simulink model "Assignment1"  (R2020a)
settings: Solver=FixedStepAuto  StartTime=0.0  StopTime=3  FixedStep=1e-3  RelTol=1e-3  EnableMultiTasking=on
undefined symbols (not defined in the file): D0, D1, D10, D11, D12, D13, D2, D3, D4, D5, D6, D7, D8, D9, PTA0, PTA1, PTA2, PTB23, PTB9, PTC16, PTC17, PTC2, PTC3, PTC4, PTD0, PTD1, PTD2, PTD3
libraries: frdmk64flib x19
settings Model: ExtModeTrigDuration=5  Creator=theodor  LastModifiedBy=theodor
settings OptimizationCC: EnhancedBackFolding=on  PassReuseOutputArgsAs=Individual arguments  ZeroExternalMemoryAtStartup=off  ZeroInternalMemoryAtStartup=off  MaxStackSize=64  OptimizeBlockOrder=speed  DifferentSizesBufferReuse=on  OptimizationCustomize=off  EfficientTunableParamExpr=on
settings DebuggingCC: ParameterTunabilityLossMsg=error
settings HardwareCC: ProdBitPerPointer=32  ProdBitPerSizeT=32  ProdBitPerPtrDiffT=32  ProdLargestAtomicInteger=Long  ProdLargestAtomicFloat=Double  ProdWordSize=32  ProdHWDeviceType=ARM Compatible->ARM Cortex
settings SFSimCC: MATLABDynamicMemAlloc=off
settings RTWCC: SystemTargetFile=ert.tlc  HardwareBoard=NXP FRDM-K64F  TemplateMakefile=ert_default_tmf  Toolchain=GNU Tools for ARM Embedded Processors
settings CodeAppCC: ForceParamTrailComments=on  IgnoreCustomStorageClasses=off  OperatorAnnotations=on  SimulinkDataObjDesc=on  SFDataObjDesc=on  InsertBlockDesc=on

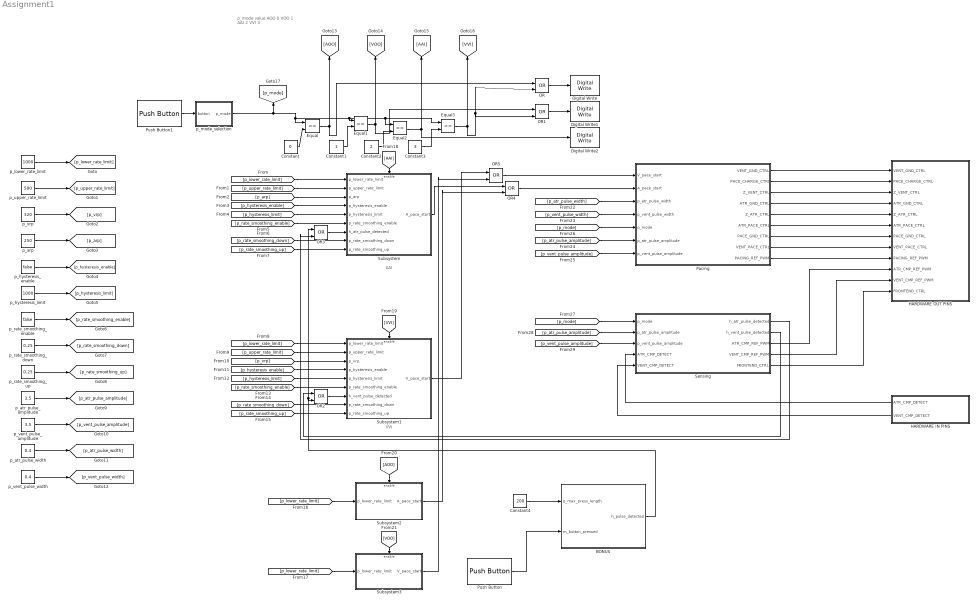
== system Assignment1 ==
  note: VVI
  note: AAI
  note: p_mode
      | value
      |
      | AOO
      | 0
      |
      | VOO
      | 1
      |
      | AAI
      | 2
      |
      | VVI
      | 3
  BONUS : Stateflow chart  TreatAsAtomicUnit=on
  Constant : Constant  Value=0
  Constant1 : Constant
  Constant2 : Constant  Value=2
  Constant3 : Constant  Value=3
  Constant4 : Constant  Value=200
  Digital Write : frdmk64flib/Digital Write  Whichpin=RED_LED
  Digital Write1 : frdmk64flib/Digital Write  Whichpin=GREEN_LED
  Digital Write2 : frdmk64flib/Digital Write  Whichpin=BLUE_LED
  Equal{,1..3} (4 alike) : RelationalOperator  Operator===  OutDataTypeStr=boolean  RndMeth=Simplest
  HARDWARE IN PINS : Subsystem
  HARDWARE OUT PINS : Subsystem
  OR{,1..5} (6 alike) : Logic  Operator=OR  IconShape=distinctive  AllPortsSameDT=off  OutDataTypeStr=boolean
  Pacing : Subsystem
  Push Button : frdmk64flib/Push Button  Whichswitch=SW3  SampleTime1=-1
  Push Button1 : frdmk64flib/Push Button  Whichswitch=SW2  SampleTime1=-1
  Sensing : Subsystem
  Subsystem : Subsystem
  Subsystem1 : Subsystem
  Subsystem2 : Subsystem
  Subsystem3 : Subsystem
  p_arp : Constant  Value=250
  p_atr_pulse_amplitude : Constant  Value=3.5
  p_atr_pulse_width : Constant  Value=0.4
  p_hysteresis_enable : Constant  Value=false
  p_hysteresis_limit : Constant  Value=1000
  p_lower_rate_limit : Constant  Value=1000
  p_mode_selection : Stateflow chart  TreatAsAtomicUnit=on
  p_rate_smoothing_down : Constant  Value=0.25
  p_rate_smoothing_enable : Constant  Value=false
  p_rate_smoothing_up : Constant  Value=0.25
  p_upper_rate_limit : Constant  Value=500
  p_vent_pulse_amplitude : Constant  Value=3.5
  p_vent_pulse_width : Constant  Value=0.4
  p_vrp : Constant  Value=320
  wires:
  Pacing/1(VENT_GND_CTRL) -> HARDWARE OUT PINS/1(VENT_GND_CTRL)
  Pacing/2(PACE_CHARGE_CTRL) -> HARDWARE OUT PINS/2(PACE_CHARGE_CTRL)
  Pacing/3(Z_VENT_CTRL) -> HARDWARE OUT PINS/3(Z_VENT_CTRL)
  Pacing/4(ATR_GND_CTRL) -> HARDWARE OUT PINS/4(ATR_GND_CTRL)
  Pacing/5(Z_ATR_CTRL) -> HARDWARE OUT PINS/5(Z_ATR_CTRL)
  Pacing/6(ATR_PACE_CTRL) -> HARDWARE OUT PINS/6(ATR_PACE_CTRL)
  Pacing/7(PACE_GND_CTRL) -> HARDWARE OUT PINS/7(PACE_GND_CTRL)
  Pacing/8(VENT_PACE_CTRL) -> HARDWARE OUT PINS/8(VENT_PACE_CTRL)
  Pacing/9(PACING_REF_PWM) -> HARDWARE OUT PINS/9(PACING_REF_PWM)
  Sensing/5(FRONTEND_CTRL) -> HARDWARE OUT PINS/12(FRONTEND_CTRL)
  Sensing/4(VENT_CMP_REF_PWM) -> HARDWARE OUT PINS/11(VENT_CMP_REF_PWM)
  Sensing/3(ATR_CMP_REF_PWM) -> HARDWARE OUT PINS/10(ATR_CMP_REF_PWM)
  HARDWARE IN PINS/1(ATR_CMP_DETECT) -> Sensing/4(ATR_CMP_DETECT)
  HARDWARE IN PINS/2(VENT_CMP_DETECT) -> Sensing/5(VENT_CMP_DETECT)
  p_mode_selection/1(p_mode) -> [p_mode], Equal3/1, Equal2/1, Equal1/1, Equal/1
  Sensing/1(h_atr_pulse_detected) -> OR3/2
  Subsystem/1(A_pace_start) -> OR4/1
  Constant/1 -> Equal/2
  Constant1/1 -> Equal1/2
  Constant2/1 -> Equal2/2
  Constant3/1 -> Equal3/2
  Equal2/1 -> Digital Write2/1, [AAI]
  Sensing/2(h_vent_pulse_detected) -> OR2/1
  Equal3/1 -> OR1/2, OR/2, [VVI]
  Equal/1 -> OR/1, [AOO]
  Equal1/1 -> OR1/1, [VOO]
  OR1/1 -> Digital Write1/1
  OR/1 -> Digital Write/1
  Push Button/1 -> BONUS/2(m_button_pressed)
  OR2/1 -> Subsystem1/7(h_vent_pulse_detected)
  BONUS/1(h_pulse_detected) -> OR3/1, OR2/2
  OR3/1 -> Subsystem/7(h_atr_pulse_detected)
  Constant4/1 -> BONUS/1(p_max_press_length)
  Push Button1/1 -> p_mode_selection/1(button)
  Subsystem2/1(A_pace_start) -> OR4/2
  OR4/1 -> Pacing/2(A_pace_start)
  Subsystem1/1(V_pace_start) -> OR5/1
  Subsystem3/1(V_pace_start) -> OR5/2
  OR5/1 -> Pacing/1(V_pace_start)
  p_lower_rate_limit/1 -> [p_lower_rate_limit]
  p_vent_pulse_width/1 -> [p_vent_pulse_width]
  p_atr_pulse_width/1 -> [p_atr_pulse_width]
  p_vent_pulse_amplitude/1 -> [p_vent_pulse_amplitude]
  p_atr_pulse_amplitude/1 -> [p_atr_pulse_amplitude]
  p_rate_smoothing_up/1 -> [p_rate_smoothing_up]
  p_rate_smoothing_down/1 -> [p_rate_smoothing_down]
  p_rate_smoothing_enable/1 -> [p_rate_smoothing_enable]
  p_hysteresis_limit/1 -> [p_hysteresis_limit]
  p_hysteresis_enable/1 -> [p_hysteresis_enable]
  p_arp/1 -> [p_arp]
  p_vrp/1 -> [p_vrp]
  p_upper_rate_limit/1 -> [p_upper_rate_limit]
  [p_lower_rate_limit] -> Subsystem/1(p_lower_rate_limit)
  [p_upper_rate_limit] -> Subsystem/2(p_upper_rate_limit)
  [p_arp] -> Subsystem/3(p_arp)
  [p_hysteresis_enable] -> Subsystem/4(p_hysteresis_enable)
  [p_hysteresis_limit] -> Subsystem/5(p_hysteresis_limit)
  [p_rate_smoothing_enable] -> Subsystem/6(p_rate_smoothing_enable)
  [p_rate_smoothing_down] -> Subsystem/8(p_rate_smoothing_down)
  [p_rate_smoothing_up] -> Subsystem/9(p_rate_smoothing_up)
  [p_lower_rate_limit] -> Subsystem1/1(p_lower_rate_limit)
  [p_upper_rate_limit] -> Subsystem1/2(p_upper_rate_limit)
  [p_vrp] -> Subsystem1/3(p_vrp)
  [p_hysteresis_enable] -> Subsystem1/4(p_hysteresis_enable)
  [p_hysteresis_limit] -> Subsystem1/5(p_hysteresis_limit)
  [p_rate_smoothing_enable] -> Subsystem1/6(p_rate_smoothing_enable)
  [p_rate_smoothing_down] -> Subsystem1/8(p_rate_smoothing_down)
  [p_rate_smoothing_up] -> Subsystem1/9(p_rate_smoothing_up)
  [p_lower_rate_limit] -> Subsystem2/1(p_lower_rate_limit)
  [p_lower_rate_limit] -> Subsystem3/1(p_lower_rate_limit)
  [AAI] -> Subsystem/Enable
  [VVI] -> Subsystem1/Enable
  [AOO] -> Subsystem2/Enable
  [VOO] -> Subsystem3/Enable
  [p_atr_pulse_width] -> Pacing/3(p_atr_pulse_width)
  [p_atr_pulse_amplitude] -> Pacing/6(p_atr_pulse_amplitude)
  [p_vent_pulse_amplitude] -> Pacing/7(p_vent_pulse_amplitude)
  [p_vent_pulse_width] -> Pacing/4(p_vent_pulse_width)
  [p_mode] -> Sensing/1(p_mode)
  [p_mode] -> Pacing/5(p_mode)
  [p_atr_pulse_amplitude] -> Sensing/2(p_atr_pulse_amplitude)
  [p_vent_pulse_amplitude] -> Sensing/3(p_vent_pulse_amplitude)

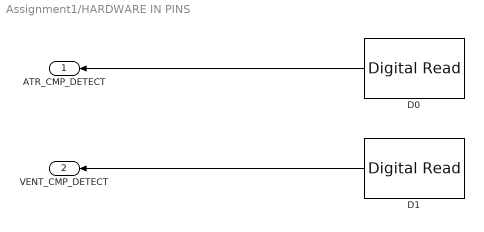
== system Assignment1/HARDWARE IN PINS ==
  D0 : frdmk64flib/Digital Read  Whichpin=PTC16 (D0)  SampleTime=-1
  D1 : frdmk64flib/Digital Read  Whichpin=PTC17 (D1)  SampleTime=-1
  ATR_CMP_DETECT : Outport
  VENT_CMP_DETECT : Outport  Port=2
  wires:
  D1/1 -> VENT_CMP_DETECT/1
  D0/1 -> ATR_CMP_DETECT/1

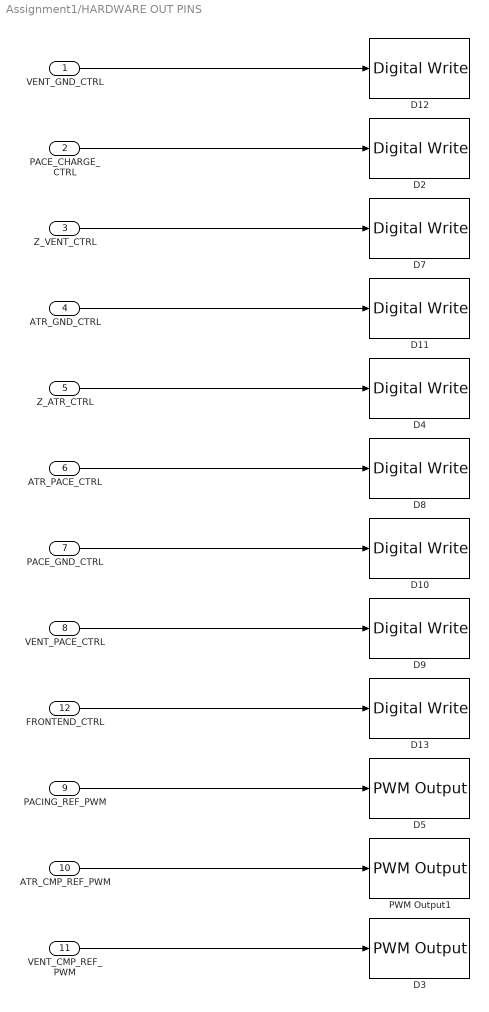
== system Assignment1/HARDWARE OUT PINS ==
  VENT_GND_CTRL : Inport
  PACE_CHARGE_CTRL : Inport  Port=2
  Z_VENT_CTRL : Inport  Port=3
  ATR_GND_CTRL : Inport  Port=4
  Z_ATR_CTRL : Inport  Port=5
  ATR_PACE_CTRL : Inport  Port=6
  PACE_GND_CTRL : Inport  Port=7
  VENT_PACE_CTRL : Inport  Port=8
  PACING_REF_PWM : Inport  Port=9
  ATR_CMP_REF_PWM : Inport  Port=10
  VENT_CMP_REF_PWM : Inport  Port=11
  FRONTEND_CTRL : Inport  Port=12
  D10 : frdmk64flib/Digital Write  Whichpin=PTD0 (D10)
  D11 : frdmk64flib/Digital Write  Whichpin=PTD2 (D11)
  D12 : frdmk64flib/Digital Write  Whichpin=PTD3 (D12)
  D13 : frdmk64flib/Digital Write  Whichpin=PTD1 (D13)
  D2 : frdmk64flib/Digital Write  Whichpin=PTB9 (D2)
  D3 : frdmk64flib/PWM Output  Whichpin=PTA1 (D3)  InitialFrequency=2000  InitialDutyCycle=0
  D4 : frdmk64flib/Digital Write  Whichpin=PTB23 (D4)
  D5 : frdmk64flib/PWM Output  Whichpin=PTA2 (D5)  InitialFrequency=2000  InitialDutyCycle=0
  D7 : frdmk64flib/Digital Write  Whichpin=PTC3 (D7)
  D8 : frdmk64flib/Digital Write  Whichpin=PTA0 (D8)
  D9 : frdmk64flib/Digital Write  Whichpin=PTC4 (D9)
  PWM Output1 : frdmk64flib/PWM Output  Whichpin=PTC2 (D6)  InitialFrequency=2000  InitialDutyCycle=0
  wires:
  ATR_PACE_CTRL/1 -> D8/1
  Z_ATR_CTRL/1 -> D4/1
  VENT_GND_CTRL/1 -> D12/1
  PACE_CHARGE_CTRL/1 -> D2/1
  FRONTEND_CTRL/1 -> D13/1
  ATR_GND_CTRL/1 -> D11/1
  PACE_GND_CTRL/1 -> D10/1
  VENT_PACE_CTRL/1 -> D9/1
  Z_VENT_CTRL/1 -> D7/1
  PACING_REF_PWM/1 -> D5/1
  ATR_CMP_REF_PWM/1 -> PWM Output1/1
  VENT_CMP_REF_PWM/1 -> D3/1

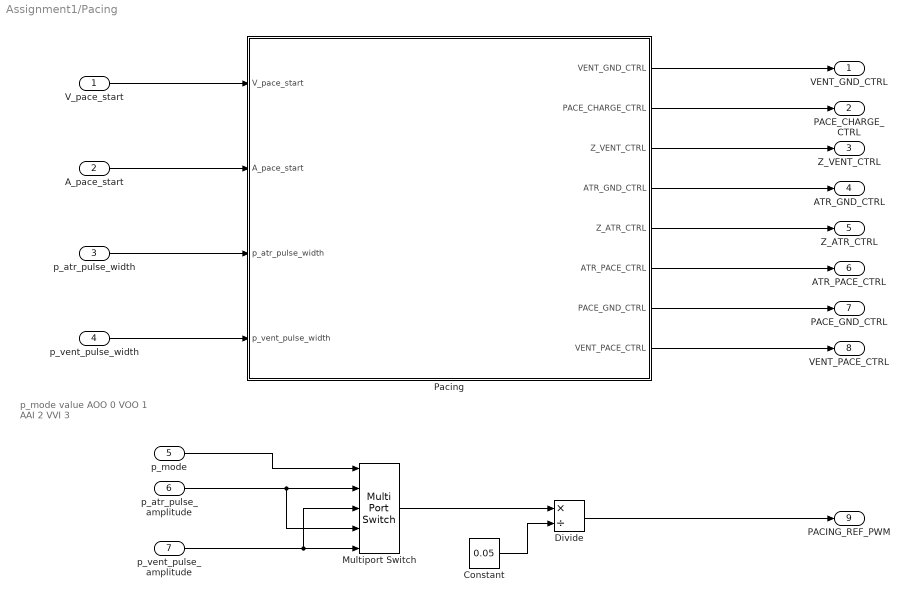
== system Assignment1/Pacing ==
  note: p_mode
      | value
      |
      | AOO
      | 0
      |
      | VOO
      | 1
      |
      | AAI
      | 2
      |
      | VVI
      | 3
  V_pace_start : Inport
  A_pace_start : Inport  Port=2
  p_atr_pulse_width : Inport  Port=3
  p_vent_pulse_width : Inport  Port=4
  p_mode : Inport  Port=5
  p_atr_pulse_amplitude : Inport  Port=6
  p_vent_pulse_amplitude : Inport  Port=7
  Constant : Constant  Value=0.05
  Divide : Product  Inputs=*/
  Multiport Switch : MultiPortSwitch  DataPortOrder=Zero-based contiguous  Inputs=4  zeroidx=on
  Pacing : Stateflow chart  TreatAsAtomicUnit=on
  VENT_GND_CTRL : Outport
  PACE_CHARGE_CTRL : Outport  Port=2
  Z_VENT_CTRL : Outport  Port=3
  ATR_GND_CTRL : Outport  Port=4
  Z_ATR_CTRL : Outport  Port=5
  ATR_PACE_CTRL : Outport  Port=6
  PACE_GND_CTRL : Outport  Port=7
  VENT_PACE_CTRL : Outport  Port=8
  PACING_REF_PWM : Outport  Port=9
  wires:
  Pacing/3(Z_VENT_CTRL) -> Z_VENT_CTRL/1
  Pacing/6(ATR_PACE_CTRL) -> ATR_PACE_CTRL/1
  A_pace_start/1 -> Pacing/2(A_pace_start)
  Pacing/5(Z_ATR_CTRL) -> Z_ATR_CTRL/1
  Pacing/2(PACE_CHARGE_CTRL) -> PACE_CHARGE_CTRL/1
  Pacing/7(PACE_GND_CTRL) -> PACE_GND_CTRL/1
  Pacing/8(VENT_PACE_CTRL) -> VENT_PACE_CTRL/1
  Pacing/4(ATR_GND_CTRL) -> ATR_GND_CTRL/1
  V_pace_start/1 -> Pacing/1(V_pace_start)
  Pacing/1(VENT_GND_CTRL) -> VENT_GND_CTRL/1
  p_mode/1 -> Multiport Switch/1
  p_atr_pulse_amplitude/1 -> Multiport Switch/4, Multiport Switch/2
  p_vent_pulse_amplitude/1 -> Multiport Switch/3, Multiport Switch/5
  Multiport Switch/1 -> Divide/1
  Constant/1 -> Divide/2
  Divide/1 -> PACING_REF_PWM/1
  p_atr_pulse_width/1 -> Pacing/3(p_atr_pulse_width)
  p_vent_pulse_width/1 -> Pacing/4(p_vent_pulse_width)

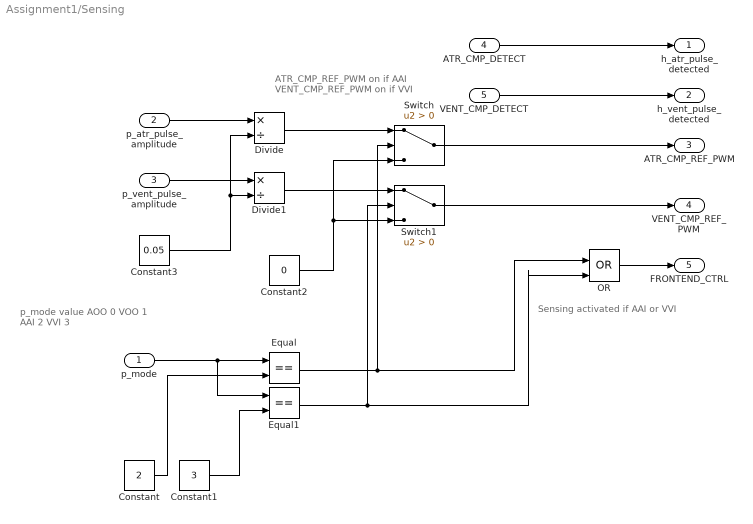
== system Assignment1/Sensing ==
  note: ATR_CMP_REF_PWM on if AAI
      | VENT_CMP_REF_PWM on if VVI
  note: Sensing activated if AAI or VVI
  note: p_mode
      | value
      |
      | AOO
      | 0
      |
      | VOO
      | 1
      |
      | AAI
      | 2
      |
      | VVI
      | 3
  p_mode : Inport
  p_atr_pulse_amplitude : Inport  Port=2
  p_vent_pulse_amplitude : Inport  Port=3
  ATR_CMP_DETECT : Inport  Port=4
  VENT_CMP_DETECT : Inport  Port=5
  Constant : Constant  Value=2
  Constant1 : Constant  Value=3
  Constant2 : Constant  Value=0
  Constant3 : Constant  Value=0.05
  Divide : Product  Inputs=*/
  Divide1 : Product  Inputs=*/
  Equal : RelationalOperator  Operator===  OutDataTypeStr=boolean  RndMeth=Simplest
  Equal1 : RelationalOperator  Operator===  OutDataTypeStr=boolean  RndMeth=Simplest
  OR : Logic  Operator=OR  IconShape=distinctive  AllPortsSameDT=off  OutDataTypeStr=boolean
  Switch : Switch  Criteria=u2 > Threshold
  Switch1 : Switch  Criteria=u2 > Threshold
  h_atr_pulse_detected : Outport
  h_vent_pulse_detected : Outport  Port=2
  ATR_CMP_REF_PWM : Outport  Port=3
  VENT_CMP_REF_PWM : Outport  Port=4
  FRONTEND_CTRL : Outport  Port=5
  wires:
  OR/1 -> FRONTEND_CTRL/1
  Equal1/1 -> Switch1/2, OR/2
  Equal/1 -> Switch/2, OR/1
  Constant/1 -> Equal/2
  Constant1/1 -> Equal1/2
  p_mode/1 -> Equal1/1, Equal/1
  Switch/1 -> ATR_CMP_REF_PWM/1
  Switch1/1 -> VENT_CMP_REF_PWM/1
  ATR_CMP_DETECT/1 -> h_atr_pulse_detected/1
  VENT_CMP_DETECT/1 -> h_vent_pulse_detected/1
  Constant2/1 -> Switch/3, Switch1/3
  p_atr_pulse_amplitude/1 -> Divide/1
  Divide/1 -> Switch/1
  Divide1/1 -> Switch1/1
  p_vent_pulse_amplitude/1 -> Divide1/1
  Constant3/1 -> Divide1/2, Divide/2

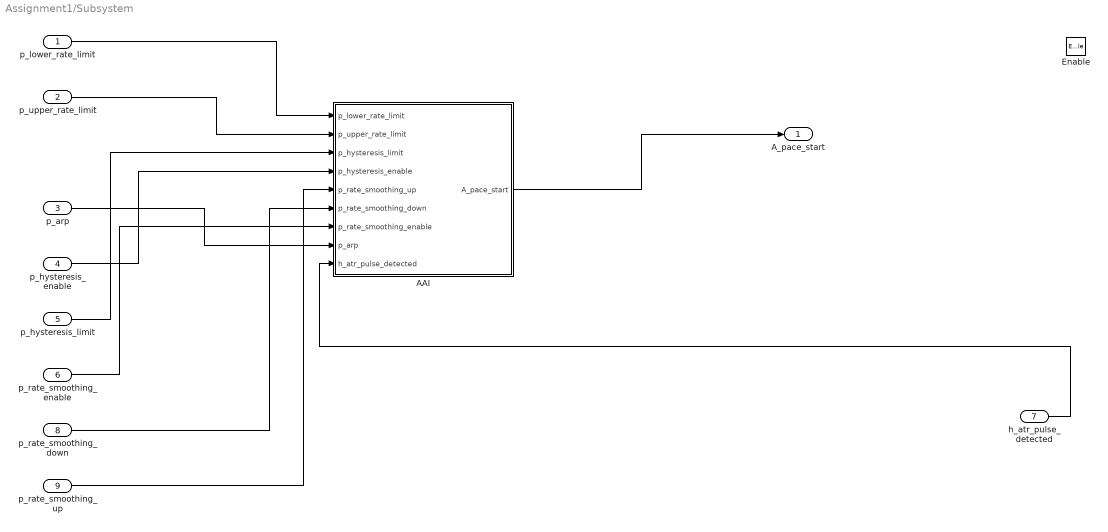
== system Assignment1/Subsystem ==
  p_lower_rate_limit : Inport
  p_upper_rate_limit : Inport  Port=2
  p_arp : Inport  Port=3
  p_hysteresis_enable : Inport  Port=4
  p_hysteresis_limit : Inport  Port=5
  p_rate_smoothing_enable : Inport  Port=6
  h_atr_pulse_detected : Inport  Port=7
  p_rate_smoothing_down : Inport  Port=8
  p_rate_smoothing_up : Inport  Port=9
  Enable : EnablePort
  AAI : Stateflow chart  TreatAsAtomicUnit=on
  A_pace_start : Outport
  wires:
  h_atr_pulse_detected/1 -> AAI/9(h_atr_pulse_detected)
  p_lower_rate_limit/1 -> AAI/1(p_lower_rate_limit)
  p_hysteresis_limit/1 -> AAI/3(p_hysteresis_limit)
  p_rate_smoothing_down/1 -> AAI/6(p_rate_smoothing_down)
  p_rate_smoothing_enable/1 -> AAI/7(p_rate_smoothing_enable)
  p_hysteresis_enable/1 -> AAI/4(p_hysteresis_enable)
  p_upper_rate_limit/1 -> AAI/2(p_upper_rate_limit)
  AAI/1(A_pace_start) -> A_pace_start/1
  p_arp/1 -> AAI/8(p_arp)
  p_rate_smoothing_up/1 -> AAI/5(p_rate_smoothing_up)

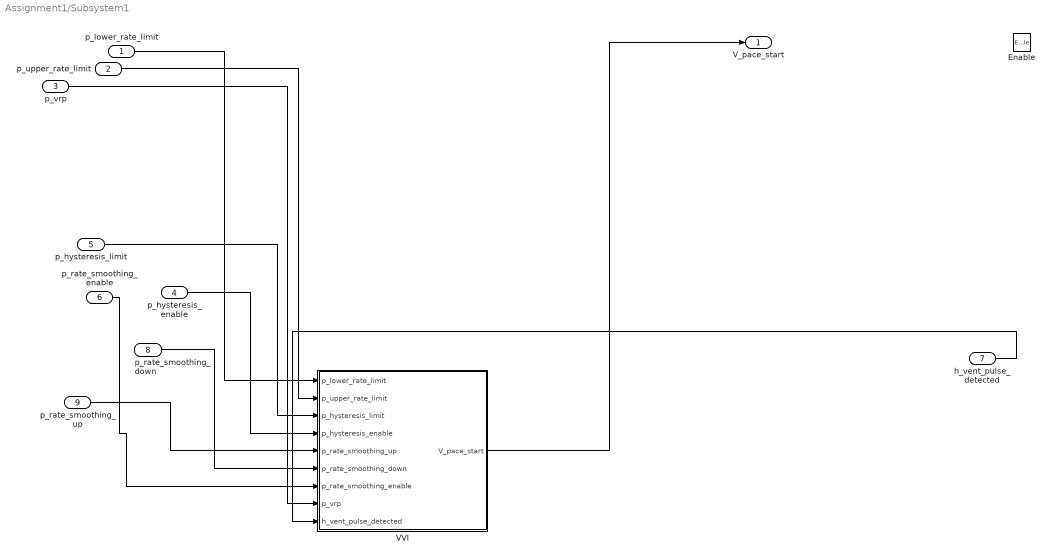
== system Assignment1/Subsystem1 ==
  p_lower_rate_limit : Inport
  p_upper_rate_limit : Inport  Port=2
  p_vrp : Inport  Port=3
  p_hysteresis_enable : Inport  Port=4
  p_hysteresis_limit : Inport  Port=5
  p_rate_smoothing_enable : Inport  Port=6
  h_vent_pulse_detected : Inport  Port=7
  p_rate_smoothing_down : Inport  Port=8
  p_rate_smoothing_up : Inport  Port=9
  Enable : EnablePort
  VVI : Stateflow chart  TreatAsAtomicUnit=on
  V_pace_start : Outport
  wires:
  p_rate_smoothing_up/1 -> VVI/5(p_rate_smoothing_up)
  p_rate_smoothing_down/1 -> VVI/6(p_rate_smoothing_down)
  p_upper_rate_limit/1 -> VVI/2(p_upper_rate_limit)
  p_rate_smoothing_enable/1 -> VVI/7(p_rate_smoothing_enable)
  p_vrp/1 -> VVI/8(p_vrp)
  p_lower_rate_limit/1 -> VVI/1(p_lower_rate_limit)
  p_hysteresis_limit/1 -> VVI/3(p_hysteresis_limit)
  h_vent_pulse_detected/1 -> VVI/9(h_vent_pulse_detected)
  VVI/1(V_pace_start) -> V_pace_start/1
  p_hysteresis_enable/1 -> VVI/4(p_hysteresis_enable)

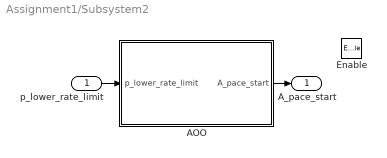
== system Assignment1/Subsystem2 ==
  p_lower_rate_limit : Inport
  Enable : EnablePort
  AOO : Stateflow chart  TreatAsAtomicUnit=on
  A_pace_start : Outport
  wires:
  p_lower_rate_limit/1 -> AOO/1(p_lower_rate_limit)
  AOO/1(A_pace_start) -> A_pace_start/1

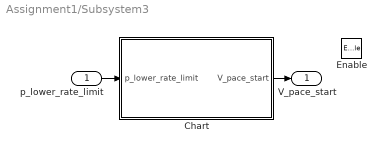
== system Assignment1/Subsystem3 ==
  p_lower_rate_limit : Inport
  Enable : EnablePort
  Chart : Stateflow chart  TreatAsAtomicUnit=on
  V_pace_start : Outport
  wires:
  p_lower_rate_limit/1 -> Chart/1(p_lower_rate_limit)
  Chart/1(V_pace_start) -> V_pace_start/1

== stateflow chart Assignment1/Subsystem/AAI ==
  state UPPER_RATE_LIMIT
    entry:
    i_limit = p_upper_rate_limit;
    i_limit = i_limit - p_arp;
    exit: i_last_period = p_arp + elapsed(msec);
  state SENSED
  state LOWER_RATE_LIMIT
    entry:
    i_limit = p_lower_rate_limit;
    i_limit = i_limit - p_arp;
    exit: i_last_period = p_arp + elapsed(msec);
  state INITIAL
    entry:
    i_limit = i_last_period;
  state HYSTERESIS_LIMIT
    entry:
    i_limit = p_hysteresis_limit;
    i_limit = i_limit - p_arp;
    exit: i_last_period = p_arp + elapsed(msec);
  state RATE_SMOOTHING_DOWN
    entry:
    i_limit = i_last_period/(1-p_rate_smoothing_down);
    i_limit = i_limit - p_arp;
    exit: i_last_period = p_arp + elapsed(msec);
  state PACED
    entry:
    A_pace_start = true;
    on after(1,msec):
    A_pace_start = false;
  state RATE_SMOOTHING_UP
    entry:
    i_limit =  i_last_period/(1+p_rate_smoothing_up);
    i_limit = i_limit - p_arp;
    exit: i_last_period = p_arp + elapsed(msec);
  (junction 89) -> SENSED
  (junction 161) -> (junction 164)
  (junction 151) -> (junction 161) [order 2]
  (junction 164) -> (junction 163)
  (junction 151) -> (junction 158) [order 1] : [p_rate_smoothing_enable]
  (junction 118) -> (junction 151) [order 1] : [p_hysteresis_enable]
  (junction 158) -> (junction 182)
  UPPER_RATE_LIMIT -> (junction 89) [order 1] : [h_atr_pulse_detected]
  (junction 182) -> (junction 184) [order 1] : [i_last_period < p_upper_rate_limit*(1-p_rate_smoothing_down)]
  (junction 184) -> UPPER_RATE_LIMIT
  (junction 88) -> (junction 89)
  (junction 182) -> (junction 168) [order 2]
  (junction 202) -> (junction 184)
  SENSED -> (junction 118) : after(p_arp, msec)
  (junction 118) -> (junction 154) [order 2]
  UPPER_RATE_LIMIT -> (junction 100) [order 2] : after(i_limit, msec)
  (default) -> (junction 193)
  INITIAL -> SENSED [order 2] : [h_atr_pulse_detected]
  (junction 100) -> (junction 101)
  (junction 168) -> (junction 170) [order 1] : [i_last_period < p_hysteresis_limit*(1-p_rate_smoothing_down)]
  (junction 168) -> (junction 187) [order 2]
  (junction 170) -> (junction 173)
  (junction 193) -> INITIAL [order 2] : {i_last_period=p_lower_rate_limit}
  (junction 193) -> INITIAL [order 1] : [p_hysteresis_enable]{i_last_period = p_hysteresis_limit}
  LOWER_RATE_LIMIT -> (junction 88) [order 1] : [h_atr_pulse_detected]
  (junction 87) -> (junction 88)
  (junction 148) -> (junction 144)
  (junction 144) -> LOWER_RATE_LIMIT
  (junction 125) -> (junction 148) [order 2]
  (junction 142) -> (junction 144)
  LOWER_RATE_LIMIT -> (junction 101) [order 2] : after(i_limit, msec)
  (junction 101) -> (junction 102)
  INITIAL -> PACED [order 1] : after(i_limit, msec)
  HYSTERESIS_LIMIT -> (junction 87) [order 1] : [h_atr_pulse_detected]
  (junction 86) -> (junction 87)
  (junction 187) -> (junction 163)
  (junction 163) -> HYSTERESIS_LIMIT
  HYSTERESIS_LIMIT -> (junction 102) [order 2] : after(i_limit, msec)
  (junction 102) -> (junction 103)
  (junction 201) -> (junction 202)
  (junction 199) -> (junction 201)
  RATE_SMOOTHING_DOWN -> (junction 86) [order 1] : [h_atr_pulse_detected]
  (junction 82) -> (junction 86)
  (junction 172) -> (junction 173)
  (junction 173) -> RATE_SMOOTHING_DOWN
  (junction 132) -> (junction 172)
  PACED -> (junction 125) : after(p_arp, msec)
  (junction 154) -> (junction 125)
  RATE_SMOOTHING_DOWN -> (junction 103) [order 2] : after(i_limit, msec)
  (junction 125) -> (junction 197) [order 1] : [p_rate_smoothing_enable]
  (junction 103) -> (junction 104)
  (junction 104) -> PACED
  (junction 197) -> (junction 199) [order 1] : [i_last_period < p_upper_rate_limit*(1-p_rate_smoothing_down)]
  (junction 197) -> (junction 128) [order 2]
  (junction 128) -> (junction 132) [order 1] : [i_last_period < p_lower_rate_limit*(1-p_rate_smoothing_down)]
  (junction 128) -> (junction 135) [order 2]
  RATE_SMOOTHING_UP -> (junction 82) [order 1] : [h_atr_pulse_detected]
  (junction 135) -> RATE_SMOOTHING_UP [order 1] : [i_last_period > p_lower_rate_limit(1+ p_rate_smoothing_up)]
  (junction 135) -> (junction 140) [order 2]
  RATE_SMOOTHING_UP -> (junction 104) [order 2] : after(i_limit, msec)
  (junction 140) -> (junction 142)
  data: p_lower_rate_limit input; p_upper_rate_limit input; p_hysteresis_limit input; p_hysteresis_enable input boolean; p_rate_smoothing_up input; p_rate_smoothing_down input; p_rate_smoothing_enable input boolean; p_arp input; i_limit local; A_pace_start output; h_atr_pulse_detected input boolean; i_last_period local

== stateflow chart Assignment1/Pacing/Pacing ==
  state Buffer
  state A_Pacing
    entry:
    PACE_CHARGE_CTRL=false;
    VENT_PACE_CTRL=false;
    VENT_GND_CTRL=false;
    ATR_GND_CTRL=false;
    ATR_PACE_CTRL=true;
  state V_Pacing
    entry:
    PACE_CHARGE_CTRL=false;
    ATR_PACE_CTRL=false;
    ATR_GND_CTRL=false;
    VENT_GND_CTRL=false;
    VENT_PACE_CTRL=true;
  state INITIAL
    entry:
    VENT_GND_CTRL=false;
    Z_VENT_CTRL=false;
    Z_ATR_CTRL=false;
    ATR_GND_CTRL=false;
  state C22_Charge
    entry:
    VENT_PACE_CTRL=false;
    ATR_PACE_CTRL=false;
    PACE_CHARGE_CTRL=true;
    PACE_GND_CTRL=true;
  state C21_Discharge_V
    entry:
    VENT_PACE_CTRL=false;
    VENT_GND_CTRL=true;
  state C21_Discharge_A
    entry:
    ATR_PACE_CTRL=false;
    ATR_GND_CTRL=true;
  Buffer -> V_Pacing [order 1] : [V_pace_start==true]
  Buffer -> A_Pacing [order 2] : [A_pace_start==true]
  C22_Charge -> Buffer : [V_pace_start==false && A_pace_start==false]
  (default) -> INITIAL
  INITIAL -> C22_Charge
  C21_Discharge_A -> C22_Charge
  C21_Discharge_V -> C22_Charge
  A_Pacing -> C21_Discharge_A : after(p_atr_pulse_width,msec)
  V_Pacing -> C21_Discharge_V : after(p_vent_pulse_width,msec)
  data: VENT_GND_CTRL output boolean; PACE_CHARGE_CTRL output boolean; Z_VENT_CTRL output boolean; ATR_GND_CTRL output boolean; Z_ATR_CTRL output boolean; ATR_PACE_CTRL output boolean; PACE_GND_CTRL output boolean; VENT_PACE_CTRL output boolean; V_pace_start input boolean; A_pace_start input boolean; p_atr_pulse_width input; p_vent_pulse_width input

== stateflow chart Assignment1/Subsystem1/VVI ==
  state UPPER_RATE_LIMIT
    entry:
    i_limit = p_upper_rate_limit;
    i_limit = i_limit - p_vrp;
    exit: i_last_period = p_vrp + elapsed(msec);
  state SENSED
  state LOWER_RATE_LIMIT
    entry:
    i_limit = p_lower_rate_limit;
    i_limit = i_limit - p_vrp;
    exit: i_last_period = p_vrp + elapsed(msec);
  state INITIAL
    entry:
    i_limit = i_last_period;
  state HYSTERESIS_LIMIT
    entry:
    i_limit = p_hysteresis_limit;
    i_limit = i_limit - p_vrp;
    exit: i_last_period = p_vrp + elapsed(msec);
  state RATE_SMOOTHING_DOWN
    entry:
    i_limit = i_last_period/(1-p_rate_smoothing_down);
    i_limit = i_limit - p_vrp;
    exit: i_last_period = p_vrp + elapsed(msec);
  state PACED
    entry:
    V_pace_start = true;
    on after(1,msec):
    V_pace_start = false;
  state RATE_SMOOTHING_UP
    entry:
    i_limit =  i_last_period/(1+p_rate_smoothing_up);
    i_limit = i_limit - p_vrp;
    exit: i_last_period = p_vrp + elapsed(msec);
  (junction 89) -> SENSED
  (junction 161) -> (junction 164)
  (junction 151) -> (junction 161) [order 2]
  (junction 164) -> (junction 163)
  (junction 151) -> (junction 158) [order 1] : [p_rate_smoothing_enable]
  (junction 118) -> (junction 151) [order 1] : [p_hysteresis_enable]
  (junction 158) -> (junction 182)
  UPPER_RATE_LIMIT -> (junction 89) [order 1] : [h_vent_pulse_detected]
  (junction 182) -> (junction 184) [order 1] : [i_last_period < p_upper_rate_limit*(1-p_rate_smoothing_down)]
  (junction 184) -> UPPER_RATE_LIMIT
  (junction 88) -> (junction 89)
  (junction 182) -> (junction 168) [order 2]
  (junction 202) -> (junction 184)
  SENSED -> (junction 118) : after(p_vrp, msec)
  (junction 118) -> (junction 154) [order 2]
  UPPER_RATE_LIMIT -> (junction 100) [order 2] : after(i_limit, msec)
  (default) -> (junction 193)
  INITIAL -> SENSED [order 2] : [h_vent_pulse_detected]
  (junction 100) -> (junction 101)
  (junction 168) -> (junction 170) [order 1] : [i_last_period < p_hysteresis_limit*(1-p_rate_smoothing_down)]
  (junction 168) -> (junction 187) [order 2]
  (junction 170) -> (junction 173)
  (junction 193) -> INITIAL [order 2] : {i_last_period=p_lower_rate_limit}
  (junction 193) -> INITIAL [order 1] : [p_hysteresis_enable]{i_last_period = p_hysteresis_limit}
  LOWER_RATE_LIMIT -> (junction 88) [order 1] : [h_vent_pulse_detected]
  (junction 87) -> (junction 88)
  (junction 148) -> (junction 144)
  (junction 144) -> LOWER_RATE_LIMIT
  (junction 125) -> (junction 148) [order 2]
  (junction 142) -> (junction 144)
  LOWER_RATE_LIMIT -> (junction 101) [order 2] : after(i_limit, msec)
  (junction 101) -> (junction 102)
  INITIAL -> PACED [order 1] : after(i_limit, msec)
  HYSTERESIS_LIMIT -> (junction 87) [order 1] : [h_vent_pulse_detected]
  (junction 86) -> (junction 87)
  (junction 187) -> (junction 163)
  (junction 163) -> HYSTERESIS_LIMIT
  HYSTERESIS_LIMIT -> (junction 102) [order 2] : after(i_limit, msec)
  (junction 102) -> (junction 103)
  (junction 201) -> (junction 202)
  (junction 199) -> (junction 201)
  RATE_SMOOTHING_DOWN -> (junction 86) [order 1] : [h_vent_pulse_detected]
  (junction 82) -> (junction 86)
  (junction 172) -> (junction 173)
  (junction 173) -> RATE_SMOOTHING_DOWN
  (junction 132) -> (junction 172)
  PACED -> (junction 125) : after(p_vrp, msec)
  (junction 154) -> (junction 125)
  RATE_SMOOTHING_DOWN -> (junction 103) [order 2] : after(i_limit, msec)
  (junction 125) -> (junction 197) [order 1] : [p_rate_smoothing_enable]
  (junction 103) -> (junction 104)
  (junction 104) -> PACED
  (junction 197) -> (junction 199) [order 1] : [i_last_period < p_upper_rate_limit*(1-p_rate_smoothing_down)]
  (junction 197) -> (junction 128) [order 2]
  (junction 128) -> (junction 132) [order 1] : [i_last_period < p_lower_rate_limit*(1-p_rate_smoothing_down)]
  (junction 128) -> (junction 135) [order 2]
  RATE_SMOOTHING_UP -> (junction 82) [order 1] : [h_vent_pulse_detected]
  (junction 135) -> RATE_SMOOTHING_UP [order 1] : [i_last_period > p_lower_rate_limit(1+ p_rate_smoothing_up)]
  (junction 135) -> (junction 140) [order 2]
  RATE_SMOOTHING_UP -> (junction 104) [order 2] : after(i_limit, msec)
  (junction 140) -> (junction 142)
  data: p_lower_rate_limit input; p_upper_rate_limit input; p_hysteresis_limit input; p_hysteresis_enable input boolean; p_rate_smoothing_up input; p_rate_smoothing_down input; p_rate_smoothing_enable input boolean; p_vrp input; i_limit local; V_pace_start output; h_vent_pulse_detected input boolean; i_last_period local

== stateflow chart Assignment1/BONUS ==
  state INVALID_PULSE
  state IDLE
    entry:
    h_pulse_detected = 0;
  state BUTTON_DOWN
    exit:
  state VALID_PULSE
    entry:
    h_pulse_detected = 1;
  INVALID_PULSE -> IDLE : [~m_button_pressed]
  BUTTON_DOWN -> INVALID_PULSE [order 2] : after(p_max_press_length,msec)
  (default) -> IDLE
  IDLE -> BUTTON_DOWN : [m_button_pressed]
  VALID_PULSE -> IDLE : after(1,msec)
  BUTTON_DOWN -> VALID_PULSE [order 1] : [~m_button_pressed]
  data: p_max_press_length input; h_pulse_detected output int8; m_button_pressed input boolean

== stateflow chart Assignment1/p_mode_selection ==
  state MODE_0
    entry:
    p_mode = 0
  state MODE_0_BUFFER
  state MODE_1
    entry:
    p_mode = 1
  state MODE_1_BUFFER
  state MODE_2
    entry:
    p_mode = 2
  state MODE_2_BUFFER
  state MODE_3
    entry:
    p_mode = 3
  state MODE_3_BUFFER
  (default) -> MODE_0
  MODE_3_BUFFER -> MODE_0 : [button]
  MODE_0 -> MODE_0_BUFFER : [~button]
  MODE_0_BUFFER -> MODE_1 : [button]
  MODE_1 -> MODE_1_BUFFER : [~button]
  MODE_1_BUFFER -> MODE_2 : [button]
  MODE_2 -> MODE_2_BUFFER : [~button]
  MODE_2_BUFFER -> MODE_3 : [button]
  MODE_3 -> MODE_3_BUFFER : [~button]
  data: button input; p_mode output

== stateflow chart Assignment1/Subsystem2/AOO ==
  state PACE
    entry:
    A_pace_start = true;
    on after(1, msec):
    A_pace_start = false;
  (default) -> PACE
  PACE -> PACE : after(p_lower_rate_limit,msec)
  data: p_lower_rate_limit input; A_pace_start output

== stateflow chart Assignment1/Subsystem3/Chart ==
  state PACE
    entry:
    V_pace_start = true;
    on after(1, msec):
    V_pace_start = false;
  (default) -> PACE
  PACE -> PACE : after(p_lower_rate_limit,msec)
  data: p_lower_rate_limit input; V_pace_start output
